simulink model "lab3_prepp_sim"  (R2020a)
settings: Solver=VariableStepAuto  StartTime=0.0  StopTime=30  RelTol=1e-3
values from neighbouring files (symbols this model uses):
  d = 0.2    [lab3.m]    (also in lab3_prepp.m = 2)
  h = 1    [lab3.m]    (also in lab3_prepp.m = 3)
libraries: simulink_extras x3
settings Model: Creator=David Wiman  LastModifiedBy=David Wiman

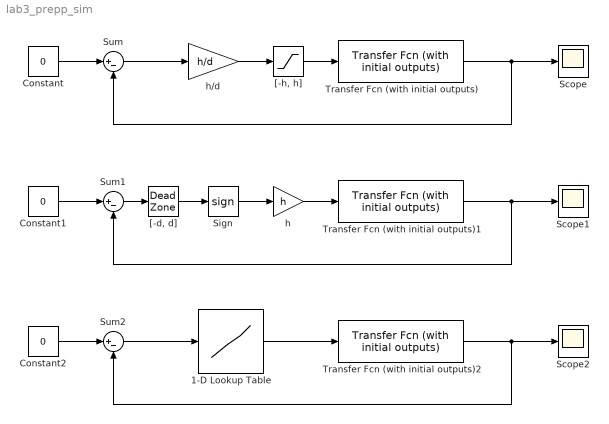
== system lab3_prepp_sim ==
  1-D Lookup Table : Lookup_n-D  NumberOfTableDimensions=1  BreakpointsForDimension1=[-1 0 1]  Table=[-0.2 0 1]  InternalRulePriority=Speed  RndMeth=Simplest  InputSameDT=on
  Constant : Constant  Value=0
  Constant1 : Constant  Value=0
  Constant2 : Constant  Value=0
  Scope : Scope
  Scope1 : Scope
  Scope2 : Scope
  Sign : Signum
  Sum : Sum  Inputs=|+-
  Sum1 : Sum  Inputs=|+-
  Sum2 : Sum  Inputs=|+-
  Transfer Fcn (with initial outputs) : simulink_extras/Additional Linear/Transfer Fcn (with initial outputs)  N=[30]  D=[1 4 7 1]  Y0=0.9132  U0=0
  Transfer Fcn (with initial outputs)1 : simulink_extras/Additional Linear/Transfer Fcn (with initial outputs)  N=[30]  D=[1 4 7 1]  Y0=0.9132  U0=0
  Transfer Fcn (with initial outputs)2 : simulink_extras/Additional Linear/Transfer Fcn (with initial outputs)  N=[30]  D=[1 4 7 1]  Y0=0.9132  U0=0
  "[-d, d]" : DeadZone  LowerValue=-d  UpperValue=d  SaturateOnIntegerOverflow=on
  "[-h, h]" : Saturate  UpperLimit=h  LowerLimit=-h
  h : Gain  Gain=h
  h/d : Gain  Gain=h/d
  wires:
  h/d/1 -> "[-h, h]"/1
  Sum/1 -> h/d/1
  Transfer Fcn (with initial outputs)/1 -> Sum/2, Scope/1
  Constant/1 -> Sum/1
  "[-h, h]"/1 -> Transfer Fcn (with initial outputs)/1
  h/1 -> Transfer Fcn (with initial outputs)1/1
  Transfer Fcn (with initial outputs)1/1 -> Sum1/2, Scope1/1
  Sum1/1 -> "[-d, d]"/1
  Constant1/1 -> Sum1/1
  "[-d, d]"/1 -> Sign/1
  Sign/1 -> h/1
  Transfer Fcn (with initial outputs)2/1 -> Sum2/2, Scope2/1
  Constant2/1 -> Sum2/1
  Sum2/1 -> 1-D Lookup Table/1
  1-D Lookup Table/1 -> Transfer Fcn (with initial outputs)2/1
